simulink model "simThreeLinkFTC"  (R2014b)
settings: Solver=ode45  StartTime=0.0  StopTime=tof  FixedStep=dt  MaxStep=dtmax  RelTol=1e-3
values from neighbouring files (symbols this model uses):
  alpha = 1    [robotArmWith2Links.m]    (also in threeLinkFTC.m; twoLinkFTC.m; twoLinkFTCwAdaptive.m)
  Ar = [0 5; -30 -30]    [robotArmWith2Links.m]    (also in threeLinkFTC.m = [0 1; -5 -5]; twoLinkFTC.m = [0 10; -40 -40]; twoLinkFTCwAdaptive.m = [0 5; -250 -250])
  Arm1 = [0 1; -wn^2 -2*ksi*wn]    [robotArmWith2Links.m]    (also in threeLinkFTC.m; twoLinkFTC.m; twoLinkFTCwAdaptive.m)
  As = zeros(nofstates,nofstates)    [threeLinkFTC.m]    (also in twoLinkFDIbasisComparison.m; twoLinkFTC.m; twoLinkFTCwAdaptive.m)
  Brm1 = [0 wn^2]'    [robotArmWith2Links.m]    (also in threeLinkFTC.m; twoLinkFTC.m; twoLinkFTCwAdaptive.m)
  Dhat0 = zeros(6,1)    [threeLinkFTC.m]    (also in twoLinkFDIbasisComparison.m = zeros(4,1); twoLinkFTC.m = zeros(4,1); twoLinkFTCwAdaptive.m = zeros(4,1))
  Dlimit = 10    [threeLinkFTC.m]    (also in twoLinkFTC.m; twoLinkFTCwAdaptive.m)
  dtFc = 1*dtmax    (= 0.001)    [threeLinkFTC.m]    (also in twoLinkFDIbasisComparison.m; twoLinkFTC.m; twoLinkFTCwAdaptive.m)
  epsilon = 0.5    [robotArmWith2Links.m]    (also in threeLinkFTC.m; twoLinkFTC.m; twoLinkFTCwAdaptive.m)
  epsilontheta = 0.01    [threeLinkFTC.m]    (also in twoLinkFDIbasisComparison.m; twoLinkFTC.m; twoLinkFTCwAdaptive.m)
  faultyArm = 3    [threeLinkFTC.m]    (also in twoLinkFDIbasisComparison.m = 2; twoLinkFTC.m = 2; twoLinkFTCwAdaptive.m = 1)
  FDstart = 0.5    [threeLinkFTC.m]    (also in twoLinkFTC.m; twoLinkFTCwAdaptive.m)
  fmPosition = [0 90 -45]'*pi/180    [threeLinkFTC.m]    (also in twoLinkFTC.m = [90 0]'*pi/180; twoLinkFTCwAdaptive.m = [90 0]'*pi/180)
  g = 9.81    [robotArmWith2Links.m]    (also in threeLinkFTC.m; twoLinkFDIbasisComparison.m; twoLinkFTC.m; twoLinkFTCwAdaptive.m)
  GammaW = 1000    [threeLinkFTC.m]    (also in twoLinkFDIbasisComparison.m; twoLinkFTC.m; twoLinkFTCwAdaptive.m)
  I1 = 8.33e-2    (= 0.0833)    [robotArmWith2Links.m]    (also in threeLinkFTC.m = 0.0833333333333; twoLinkFDIbasisComparison.m = 0.0833333333333; twoLinkFTC.m = 0.0833333333333; twoLinkFTCwAdaptive.m = 0.0833333333333)
  I2 = 8.33e-2    (= 0.0833)    [robotArmWith2Links.m]    (also in threeLinkFTC.m = 0.0833333333333; twoLinkFDIbasisComparison.m = 0.0833333333333; twoLinkFTC.m = 0.0833333333333; twoLinkFTCwAdaptive.m = 0.0833333333333)
  I3 = m3*l3^2*1/12    (= 0.0833333333333)    [threeLinkFTC.m]
  ifault = 2    [threeLinkFTC.m]    (also in twoLinkFDIbasisComparison.m; twoLinkFTC.m; twoLinkFTCwAdaptive.m)
  K1 = 2*wn*ksi    (= 87.9645943005)    [robotArmWith2Links.m]    (also in threeLinkFTC.m = 8.79645943005; twoLinkFTC.m; twoLinkFTCwAdaptive.m = 43.9822971503)
  K2 = wn^2    (= 986.960440109)    [robotArmWith2Links.m]    (also in threeLinkFTC.m = 39.4784176044; twoLinkFTC.m; twoLinkFTCwAdaptive.m)
  Kp = wn^2    (= 157.913670417)    [threeLinkFTC.m]    (also in twoLinkFDIbasisComparison.m = 3947.84176044; twoLinkFTC.m = 3947.84176044; twoLinkFTCwAdaptive.m = 3947.84176044)
  Kv = 2*ksi*wn    (= 17.5929188601)    [threeLinkFTC.m]    (also in twoLinkFDIbasisComparison.m = 125.663706144; twoLinkFTC.m = 125.663706144; twoLinkFTCwAdaptive.m = 125.663706144)
  l1 = 1    [robotArmWith2Links.m]    (also in threeLinkFTC.m; twoLinkFDIbasisComparison.m; twoLinkFTC.m; twoLinkFTCwAdaptive.m)
  l2 = 1    [robotArmWith2Links.m]    (also in threeLinkFTC.m; twoLinkFDIbasisComparison.m; twoLinkFTC.m; twoLinkFTCwAdaptive.m)
  lc1 = l1/2    (= 0.5)    [robotArmWith2Links.m]    (also in threeLinkFTC.m; twoLinkFDIbasisComparison.m; twoLinkFTC.m; twoLinkFTCwAdaptive.m)
  lc2 = l2/2    (= 0.5)    [robotArmWith2Links.m]    (also in threeLinkFTC.m; twoLinkFDIbasisComparison.m; twoLinkFTC.m; twoLinkFTCwAdaptive.m)
  m1 = 1    [robotArmWith2Links.m]    (also in threeLinkFTC.m; twoLinkFDIbasisComparison.m; twoLinkFTC.m; twoLinkFTCwAdaptive.m)
  m2 = 1    [robotArmWith2Links.m]    (also in threeLinkFTC.m; twoLinkFDIbasisComparison.m; twoLinkFTC.m; twoLinkFTCwAdaptive.m)
  m3 = 1    [threeLinkFTC.m]
  nCheby = 4    [threeLinkFTC.m]    (also in twoLinkFDIbasisComparison.m; twoLinkFTC.m; twoLinkFTCwAdaptive.m)
  Ps = lyap(As(4:6,4:6)',Q)    [threeLinkFTC.m]    (also in twoLinkFDIbasisComparison.m = lyap(As(3:4,3:4)',Q); twoLinkFTC.m = lyap(As(3:4,3:4)',Q); twoLinkFTCwAdaptive.m = lyap(As(3:4,3:4)',Q))
  q0 = [80 20]'*pi/180    [robotArmWith2Links.m]    (also in threeLinkFTC.m = [90 0 0]'*pi/180; twoLinkFDIbasisComparison.m = [90 0]'*pi/180; twoLinkFTC.m = [90 0]'*pi/180; twoLinkFTCwAdaptive.m = [90 0]'*pi/180)
  qdot0 = [0 0]'    [robotArmWith2Links.m]    (also in threeLinkFTC.m = [0 0 0]'*pi/180; twoLinkFDIbasisComparison.m = [0 0]'*pi/180; twoLinkFTC.m = [0 0]'*pi/180; twoLinkFTCwAdaptive.m = [0 0]'*pi/180)
  r0 = [0 0]'    [robotArmWith2Links.m]    (also in threeLinkFTC.m; twoLinkFTC.m; twoLinkFTCwAdaptive.m)
  rmax = inf*[50*pi/180 inf]'    [robotArmWith2Links.m]    (also in threeLinkFTC.m; twoLinkFTC.m; twoLinkFTCwAdaptive.m)
  rmin = -rmax    [robotArmWith2Links.m]    (also in threeLinkFTC.m; twoLinkFTC.m; twoLinkFTCwAdaptive.m)
  tfault = 5    [threeLinkFTC.m]    (also in twoLinkFDIbasisComparison.m; twoLinkFTC.m; twoLinkFTCwAdaptive.m = 1)
  W0 = 0    [threeLinkFTC.m]    (also in twoLinkFDIbasisComparison.m; twoLinkFTC.m; twoLinkFTCwAdaptive.m)
  Wbnd = 1000    [threeLinkFTC.m]    (also in twoLinkFDIbasisComparison.m; twoLinkFTC.m; twoLinkFTCwAdaptive.m)
  xhat0 = [q0 ; qdot0]    [threeLinkFTC.m]    (also in twoLinkFDIbasisComparison.m; twoLinkFTC.m; twoLinkFTCwAdaptive.m)
undefined symbols (not defined in the file or in its folder): Intmax, Intmin
libraries: simulink x9, vrlib x3, dspbuff3 x1
(part 1 of 3)
settings Model: Creator=alp.marangoz  LastModifiedBy=alpmarangoz
settings SolverCC: AutoInsertRateTranBlk=on
settings DataIOCC: SignalLoggingSaveFormat=ModelDataLogs
settings OptimizationCC: ExpressionDepthLimit=2147483647
settings DebuggingCC: UnderspecifiedInitializationDetection=Classic  MergeDetectMultiDrivingBlocksExec=none  InheritedTsInSrcMsg=none  CheckMatrixSingularityMsg=error  FcnCallInpInsideContextMsg=UseLocalSettings  StateNameClashWarn=warning
settings GRTTargetCC: CombineOutputUpdateFcns=off  GRTInterface=on

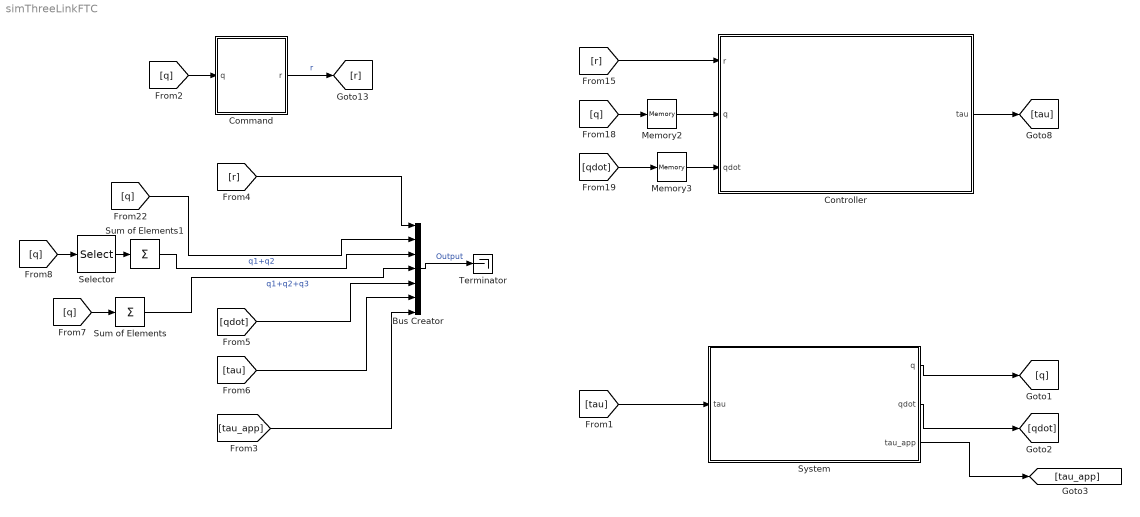
== system simThreeLinkFTC ==
  Bus Creator : BusCreator  Inputs=7
  Command : Subsystem  TreatAsAtomicUnit=on  SystemSampleTime=dtFc
  Controller : Subsystem  TreatAsAtomicUnit=on  SystemSampleTime=dtFc
  Memory2 : Memory  X0=q0  InheritSampleTime=on  LinearizeMemory=on  LinearizeAsDelay=on
  Memory3 : Memory  X0=qdot0  InheritSampleTime=on  LinearizeMemory=on  LinearizeAsDelay=on
  Selector : Selector  InputPortWidth=3  Indices=[1 2]
  Sum of Elements : Sum  Inputs=+
  Sum of Elements1 : Sum  Inputs=+
  System : Subsystem  TreatAsAtomicUnit=on
  Terminator : Terminator
  wires:
  Command/1(r) -> [r]  "r"
  [r] -> Controller/1(r)
  Controller/1(tau) -> [tau]
  [tau] -> System/1(tau)
  [q] -> Memory2/1
  [qdot] -> Memory3/1
  System/1(q) -> [q]
  System/2(qdot) -> [qdot]
  [q] -> Command/1(q)
  Memory2/1 -> Controller/2(q)
  Memory3/1 -> Controller/3(qdot)
  Bus Creator/1 -> Terminator/1  "Output"
  [r] -> Bus Creator/1
  [q] -> Bus Creator/2
  [qdot] -> Bus Creator/5
  [tau] -> Bus Creator/6
  System/3(tau_app) -> [tau_app]
  [tau_app] -> Bus Creator/7
  [q] -> Selector/1
  Selector/1 -> Sum of Elements1/1
  Sum of Elements1/1 -> Bus Creator/3  "q1+q2"
  [q] -> Sum of Elements/1
  Sum of Elements/1 -> Bus Creator/4  "q1+q2+q3"

== system simThreeLinkFTC/Command ==
  q : Inport
  Add1 : Sum  Inputs=-+
  From Workspace : FromWorkspace  VariableName=r  Interpolate=off  OutputAfterFinalValue=Setting to zero
  Memory2 : Memory  X0=q0  InheritSampleTime=on  LinearizeMemory=on  LinearizeAsDelay=on
  Reshape1 : Reshape  OutputDimensionality=Column vector (2-D)
  Terminator1 : Terminator
  r : Outport  InitialOutput=0
  wires:
  From Workspace/1 -> Reshape1/1
  Reshape1/1 -> r/1, [r]  "r"
  [r] -> Add1/2
  Add1/1 -> Terminator1/1  "e"
  [q] -> Add1/1  "q"
  q/1 -> Memory2/1  "q"
  Memory2/1 -> [q]

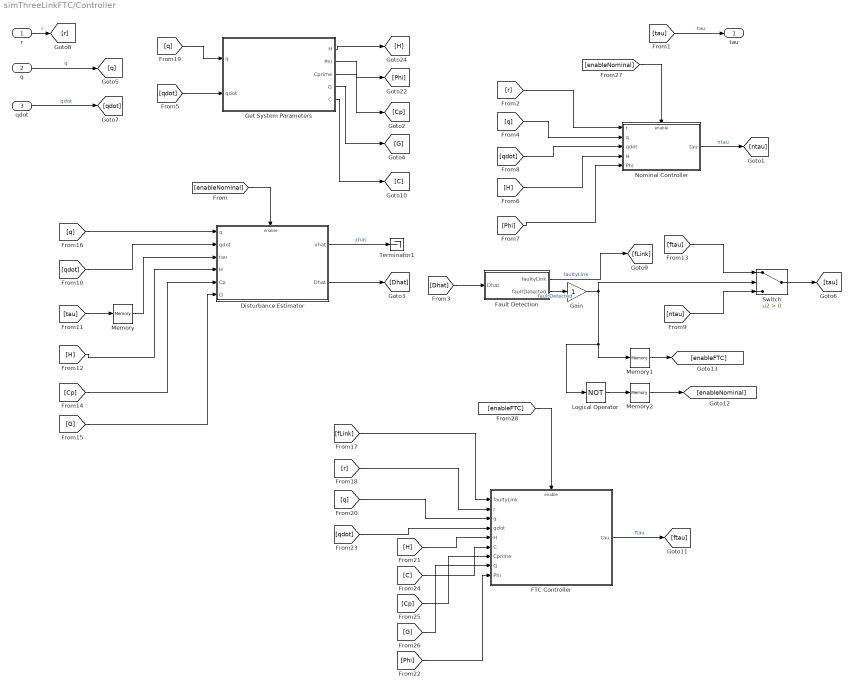
== system simThreeLinkFTC/Controller ==
  r : Inport
  q : Inport  Port=2
  qdot : Inport  Port=3
  Disturbance Estimator : Subsystem
  FTC Controller : Subsystem
  Fault Detection : Subsystem  TreatAsAtomicUnit=on
  Gain : Gain
  Get System Parameters : Subsystem
  Logical Operator : Logic  Operator=NOT  AllPortsSameDT=off  OutDataTypeStr=boolean
  Memory : Memory  InheritSampleTime=on  LinearizeMemory=on  LinearizeAsDelay=on
  Memory1 : Memory  InheritSampleTime=on  LinearizeMemory=on  LinearizeAsDelay=on
  Memory2 : Memory  InheritSampleTime=on  LinearizeMemory=on  LinearizeAsDelay=on
  Nominal Controller : Subsystem
  Switch : Switch  Criteria=u2 > Threshold
  Terminator1 : Terminator
  tau : Outport
  wires:
  r/1 -> [r]  "r"
  qdot/1 -> [qdot]  "qdot"
  q/1 -> [q]  "q"
  [tau] -> tau/1  "tau"
  [q] -> Get System Parameters/1(q)
  Nominal Controller/1(tau) -> [ntau]  "ntau"
  [r] -> Nominal Controller/1(r)
  [H] -> Nominal Controller/4(H)
  [Phi] -> Nominal Controller/5(Phi)
  [qdot] -> Get System Parameters/2(qdot)
  Get System Parameters/1(H) -> [H]
  Get System Parameters/2(Phi) -> [Phi]
  Get System Parameters/3(Cprime) -> [Cp]
  [q] -> Disturbance Estimator/1(q)
  [qdot] -> Disturbance Estimator/2(qdot)
  [H] -> Disturbance Estimator/4(H)
  [Cp] -> Disturbance Estimator/5(Cp)
  [G] -> Disturbance Estimator/6(G)
  Disturbance Estimator/1(xhat) -> Terminator1/1  "xhat"
  Disturbance Estimator/2(Dhat) -> [Dhat]
  [qdot] -> Nominal Controller/3(qdot)
  [q] -> Nominal Controller/2(q)
  [tau] -> Memory/1
  Get System Parameters/4(G) -> [G]
  [Dhat] -> Fault Detection/1(Dhat)
  Switch/1 -> [tau]
  Fault Detection/2(faultDetected) -> Gain/1  "faultDetected"
  [ntau] -> Switch/3
  [ftau] -> Switch/1
  Fault Detection/1(faultyLink) -> [fLink]  "faultyLink"
  Get System Parameters/5(C) -> [C]
  FTC Controller/1(tau) -> [ftau]  "ftau"
  [H] -> FTC Controller/5(H)
  [C] -> FTC Controller/6(C)
  [Cp] -> FTC Controller/7(Cprime)
  [G] -> FTC Controller/8(G)
  [qdot] -> FTC Controller/4(qdot)
  [q] -> FTC Controller/3(q)
  [Phi] -> FTC Controller/9(Phi)
  [r] -> FTC Controller/2(r)
  [fLink] -> FTC Controller/1(faultyLink)
  Memory/1 -> Disturbance Estimator/3(tau)
  [enableNominal] -> Disturbance Estimator/Enable
  [enableNominal] -> Nominal Controller/Enable
  Logical Operator/1 -> Memory2/1
  [enableFTC] -> FTC Controller/Enable
  Memory1/1 -> [enableFTC]
  Memory2/1 -> [enableNominal]
  Gain/1 -> Switch/2, Logical Operator/1, Memory1/1

== system simThreeLinkFTC/System ==
  tau : Inport
  Fault Insertion : Subsystem
  Integration : Subsystem  TreatAsAtomicUnit=on
  Memory2 : Memory  X0=q0  InheritSampleTime=on  LinearizeMemory=on  LinearizeAsDelay=on
  Memory4 : Memory  X0=qdot0  InheritSampleTime=on  LinearizeMemory=on  LinearizeAsDelay=on
  Reshape5 : Reshape  OutputDimensionality=Column vector (2-D)
  System Parameters : Subsystem
  q : Outport
  qdot : Outport  Port=2
  tau_app : Outport  Port=3
  wires:
  [q] -> Memory2/1
  [qdot] -> Memory4/1
  tau/1 -> Reshape5/1  "tau"
  Reshape5/1 -> [tau]  "tau"
  [q] -> q/1  "q"
  [qdot] -> qdot/1  "qdot"
  Memory4/1 -> System Parameters/2(qdot)
  [H] -> Integration/1(H)
  [C] -> Integration/2(C)
  [tau_app] -> Integration/4(tau)
  [lockJoint] -> Integration/5(lockJoint)
  [G] -> Integration/3(G)
  Integration/1(q) -> [q]
  Integration/2(qdot) -> [qdot]
  Memory2/1 -> System Parameters/1(q)
  Fault Insertion/2(lockJoint) -> [lockJoint]
  Fault Insertion/1(tau_app) -> [tau_app]
  [tau] -> Fault Insertion/1(tau)
  [tau_app] -> tau_app/1  "tau_app"
  System Parameters/1(H) -> [H]
  System Parameters/2(C) -> [C]
  System Parameters/3(G) -> [G]

== system simThreeLinkFTC/Controller/Disturbance Estimator ==
  q : Inport
  qdot : Inport  Port=2
  tau : Inport  Port=3
  H : Inport  Port=4
  Cp : Inport  Port=5
  G : Inport  Port=6
  Enable : EnablePort
  Memory1 : Memory  X0=Dhat0  InheritSampleTime=on  LinearizeMemory=on
  Product3 : Product  Inputs=/  Multiplication=Matrix(*)  RndMeth=Zero
  State Error Calculation : Subsystem
  getDisturbance : Subsystem
  getx : Subsystem
  getxhat : Subsystem
  xhat : Outport  InitialOutput=xhat0
  Dhat : Outport  Port=2
  wires:
  getx/2(xdot) -> [xdot]
  [qdot] -> getx/2(qdot)
  [q] -> getx/1(q)
  Cp/1 -> [Cp]
  Product3/1 -> [Hinv]
  H/1 -> [H], Product3/1
  tau/1 -> [tau]
  [xhat] -> xhat/1
  q/1 -> [q]
  qdot/1 -> [qdot]
  getx/1(x) -> [x]  "x"
  [H] -> getx/3(H)
  [Hinv] -> getxhat/1(Hinv)
  [tau] -> getxhat/2(tau)
  [Cp] -> getxhat/3(Cp)
  [es] -> getxhat/5(es)
  [Dhat] -> Memory1/1
  G/1 -> [G]
  getxhat/1(xhat) -> [xhat]  "xhat"
  getxhat/2(xhatdot) -> [xhatdot]
  [x] -> State Error Calculation/1(x)
  [xdot] -> State Error Calculation/2(xdot)
  [xhat] -> State Error Calculation/3(xhat)
  [xhatdot] -> State Error Calculation/4(xhatdot)
  [Hinv] -> State Error Calculation/5(Hinv)
  State Error Calculation/1(es) -> [es]
  [xhat] -> getDisturbance/1(x)
  [tau] -> getDisturbance/2(tau)
  [es] -> getDisturbance/3(es)
  getDisturbance/1(Dhat) -> [Dhat]
  [Dhat] -> Dhat/1
  Memory1/1 -> getxhat/6(Dhat)
  [G] -> getxhat/4(G)

== system simThreeLinkFTC/Controller/FTC Controller ==
  faultyLink : Inport
  r : Inport  Port=2
  q : Inport  Port=3
  qdot : Inport  Port=4
  H : Inport  Port=5
  C : Inport  Port=6
  Cprime : Inport  Port=7
  G : Inport  Port=8
  Phi : Inport  Port=9
  Enable : EnablePort
  1st Link Compensator : Subsystem  TreatAsAtomicUnit=on  SystemSampleTime=dtFc
  3rd Link Compensator : Subsystem  TreatAsAtomicUnit=on  SystemSampleTime=dtFc
  Compare To Constant : simulink/Logic and Bit Operations/Compare To Constant  relop===  const=3.0  OutDataTypeStr=boolean
  Compare To Constant1 : simulink/Logic and Bit Operations/Compare To Constant  relop===  const=1  OutDataTypeStr=boolean
  Constant : Constant  Value=fmPosition  VectorParams1D=off
  Gain1 : Gain  Gain=[1 2 3]  Multiplication=Matrix(K*u)
  Ground : Ground
  Multiport Switch : MultiPortSwitch
  Terminator1 : Terminator
  Terminator6 : Terminator
  Terminator8 : Terminator
  tau : Outport
  wires:
  [tau] -> tau/1  "tau"
  faultyLink/1 -> Gain1/1
  Cprime/1 -> Terminator6/1
  G/1 -> [G]
  Phi/1 -> Terminator8/1
  q/1 -> [q]
  qdot/1 -> [qdot]
  H/1 -> [H]
  C/1 -> [C]
  r/1 -> Terminator1/1  "r"
  Constant/1 -> [qc]
  [H] -> 3rd Link Compensator/4(H)
  [G] -> 3rd Link Compensator/6(G)
  [qdot] -> 3rd Link Compensator/3(qdot)
  [C] -> 3rd Link Compensator/5(C)
  [q] -> 3rd Link Compensator/2(q)
  [qc] -> 3rd Link Compensator/1(qc)
  [H] -> 1st Link Compensator/4(H)
  [G] -> 1st Link Compensator/6(G)
  [qdot] -> 1st Link Compensator/3(qdot)
  [C] -> 1st Link Compensator/5(C)
  [q] -> 1st Link Compensator/2(q)
  [qc] -> 1st Link Compensator/1(qc)
  3rd Link Compensator/1(tau) -> [tau_3comp]  "tau3_comp"
  1st Link Compensator/1(tau) -> [tau_1comp]  "tau1_comp"
  Multiport Switch/1 -> [tau]  "tau"
  [tau_3comp] -> Multiport Switch/4
  Ground/1 -> Multiport Switch/3
  [tau_1comp] -> Multiport Switch/2
  Gain1/1 -> [faultyArm]  "faultyArm"
  [faultyArm] -> Multiport Switch/1
  [faultyArm] -> Compare To Constant/1
  Compare To Constant/1 -> 3rd Link Compensator/Enable
  [faultyArm] -> Compare To Constant1/1
  Compare To Constant1/1 -> 1st Link Compensator/Enable

== system simThreeLinkFTC/Controller/Fault Detection ==
  Dhat : Inport
  Abs : Abs
  Compare To Constant : simulink/Logic and Bit Operations/Compare To Constant  relop=>=  const=Dlimit  OutDataTypeStr=boolean
  Compare To Constant1 : simulink/Logic and Bit Operations/Compare To Constant  relop=>=  const=FDstart  OutDataTypeStr=boolean
  Digital Clock : DigitalClock  SampleTime=-1
  Logical Operator : Logic  AllPortsSameDT=off  OutDataTypeStr=boolean
  Select 3 : Selector  NumberOfDimensions=2  InputPortWidth=3  IndexOptions=Index vector (dialog),Index vector (dialog)  Indices=[4 5 6],1  OutputSizes=1,1
  Sum of Elements : Sum  Inputs=+
  Triggered step : Subsystem
  faultyLink : Outport
  faultDetected : Outport  Port=2
  wires:
  Dhat/1 -> Select 3/1
  Abs/1 -> Compare To Constant/1
  Select 3/1 -> Abs/1
  Compare To Constant/1 -> Sum of Elements/1, faultyLink/1
  Triggered step/1(Out1) -> faultDetected/1
  Sum of Elements/1 -> Logical Operator/1
  Logical Operator/1 -> Triggered step/Trigger
  Digital Clock/1 -> Compare To Constant1/1
  Compare To Constant1/1 -> Logical Operator/2

== system simThreeLinkFTC/Controller/Get System Parameters ==
  q : Inport
  qdot : Inport  Port=2
  Constant : Constant  Value=I1+m1*lc1^2+m2*l1^2+m3*l1^2  VectorParams1D=off
  Constant2 : Constant  Value=[0 0 0]'  VectorParams1D=off
  Constant3 : Constant  Value=I2+I3+m2*lc2^2+m3*l2^2  VectorParams1D=off
  Constant4 : Constant  Value=m2*l1*lc2+m3*l1*l2  VectorParams1D=off
  Constant5 : Constant  Value=I3  VectorParams1D=off
  Product5 : Product  Multiplication=Matrix(*)  RndMeth=Zero
  Sum of Elements1 : Sum
  Terminator18 : Terminator
  get Plant Parameters : Subsystem
  getC : Subsystem
  getCprime : Subsystem
  getH : Subsystem
  H : Outport
  Phi : Outport  Port=2
  Cprime : Outport  Port=3
  G : Outport  Port=4
  C : Outport  Port=5
  wires:
  q/1 -> [q]
  qdot/1 -> [qdot]
  getH/1(H) -> [H]
  Constant2/1 -> [G]
  [C] -> Product5/1
  [qdot] -> Product5/2
  Product5/1 -> Sum of Elements1/1
  [G] -> Sum of Elements1/2
  Sum of Elements1/1 -> [Phi]  "Phi"
  [H] -> H/1
  [Phi] -> Phi/1
  [Cprime] -> Cprime/1
  Constant/1 -> [alpha]
  [G] -> G/1
  get Plant Parameters/1(busData) -> Terminator18/1  "system"
  [C] -> get Plant Parameters/2(C)
  [H] -> get Plant Parameters/1(H)
  [G] -> get Plant Parameters/3(G)
  [qdot] -> get Plant Parameters/4(qdot)
  [Cprime] -> get Plant Parameters/5(Cprime)
  [C] -> C/1
  Constant3/1 -> [beta]
  Constant4/1 -> [gamma]
  Constant5/1 -> [delta]
  [alpha] -> getH/2(alpha)
  [beta] -> getH/3(beta)
  [gamma] -> getH/4(gamma)
  [delta] -> getH/5(delta)
  [q] -> getH/1(q)
  getC/1(C) -> [C]
  [alpha] -> getC/3(alpha)
  [beta] -> getC/4(beta)
  [gamma] -> getC/5(gamma)
  [delta] -> getC/6(delta)
  [q] -> getC/1(q)
  [qdot] -> getC/2(qdot)
  getCprime/1(Cprime) -> [Cprime]
  [alpha] -> getCprime/3(alpha)
  [beta] -> getCprime/4(beta)
  [gamma] -> getCprime/5(gamma)
  [delta] -> getCprime/6(delta)
  [q] -> getCprime/1(q)
  [qdot] -> getCprime/2(qdot)

== system simThreeLinkFTC/Controller/Nominal Controller ==
  r : Inport
  q : Inport  Port=2
  qdot : Inport  Port=3
  H : Inport  Port=4
  Phi : Inport  Port=5
  Enable : EnablePort
  FBL Controller : Subsystem
  Saturation : Saturate  UpperLimit=2000  LowerLimit=-2000
  tau : Outport
  wires:
  r/1 -> [r]  "r"
  Phi/1 -> [Phi]
  H/1 -> [H]
  [tau] -> Saturation/1  "tau"
  [r] -> FBL Controller/1(r)
  [H] -> FBL Controller/4(H)
  [Phi] -> FBL Controller/5(Phi)
  Saturation/1 -> tau/1
  FBL Controller/1(tau) -> [tau]
  q/1 -> [q]
  qdot/1 -> [qdot]
  [qdot] -> FBL Controller/3(qdot)
  [q] -> FBL Controller/2(q)

== system simThreeLinkFTC/System/Fault Insertion ==
  tau : Inport
  Clock : Clock
  Compare To Constant : simulink/Logic and Bit Operations/Compare To Constant  relop===  const=faultyArm  OutDataTypeStr=boolean
  Compare To Constant1 : simulink/Logic and Bit Operations/Compare To Constant  relop===  const=3  OutDataTypeStr=uint8  ZeroCross=off
  Constant1 : Constant  Value=ifault  VectorParams1D=off
  Constant2 : Constant  Value=[ 1 1 1]'
  Constant4 : Constant  Value=tfault
  Constant5 : Constant  Value=[1 2 3]'  VectorParams1D=off
  Data Type Conversion : DataTypeConversion
  Data Type Conversion1 : DataTypeConversion
  Ground2 : Ground
  Logical Operator1 : Logic  Operator=NOT  AllPortsSameDT=off  OutDataTypeStr=boolean
  Logical Operator2 : Logic  AllPortsSameDT=off  OutDataTypeStr=boolean
  MinMax1 : MinMax  Function=max  Inputs=2
  Product : Product
  Sign : Signum
  Subtract1 : Sum  Inputs=+-
  Switch2 : Switch  Criteria=u2 > Threshold
  Switch3 : Switch  Criteria=u2 > Threshold
  tau_app : Outport
  lockJoint : Outport  Port=2
  wires:
  Clock/1 -> [time]
  MinMax1/1 -> [faultInsertion]  "faultInsertion"
  Sign/1 -> MinMax1/1
  Ground2/1 -> MinMax1/2
  Subtract1/1 -> Sign/1
  Constant4/1 -> Subtract1/2
  [time] -> Subtract1/1
  tau/1 -> [tau]  "tau"
  Constant1/1 -> Compare To Constant1/1
  Data Type Conversion1/1 -> [lockJoint]
  [faultInsertion] -> Switch2/2
  [faultytau] -> Switch2/1
  [tau] -> Switch2/3
  Switch2/1 -> tau_app/1  "tau_app"
  [faultyJoint] -> Switch3/1
  Constant2/1 -> Switch3/3
  Switch3/1 -> lockJoint/1  "lockJoint"
  Compare To Constant1/1 -> Data Type Conversion1/1
  Compare To Constant/1 -> Logical Operator1/1
  Constant5/1 -> Compare To Constant/1
  Logical Operator1/1 -> Data Type Conversion/1
  Data Type Conversion/1 -> [faultyJoint]
  Product/1 -> [faultytau]
  [faultyJoint] -> Product/1
  [tau] -> Product/2
  [faultInsertion] -> Logical Operator2/1
  [lockJoint] -> Logical Operator2/2
  Logical Operator2/1 -> Switch3/2

== system simThreeLinkFTC/System/Integration ==
  H : Inport
  C : Inport  Port=2
  G : Inport  Port=3
  tau : Inport  Port=4
  lockJoint : Inport  Port=5
  Add : Sum  Inputs=+-
  Constant1 : Constant  Value=2*pi
  Integrator2 : Integrator  InitialCondition=qdot0
  Integrator3 : Integrator  InitialCondition=q0
  Math Function1 : Math  Operator=rem  SaturateOnIntegerOverflow=on
  Product1 : Product  RndMeth=Zero
  Product3 : Product  RndMeth=Zero
  Product4 : Product  Multiplication=Matrix(*)  RndMeth=Zero
  Product5 : Product  Multiplication=Matrix(*)  RndMeth=Zero
  Product6 : Product  Multiplication=Matrix(*)  RndMeth=Zero
  Product7 : Product  Inputs=/  Multiplication=Matrix(*)  RndMeth=Zero
  Reshape : Reshape  OutputDimensionality=Column vector (2-D)
  Reshape3 : Reshape  OutputDimensionality=Column vector (2-D)
  Sum : Sum  Inputs=|+-
  q : Outport
  qdot : Outport  Port=2
  wires:
  lockJoint/1 -> [lockJoint]
  tau/1 -> [tau]
  C/1 -> [C]
  H/1 -> Product7/1
  [qdot] -> qdot/1  "qdot"
  [q] -> q/1  "q"
  G/1 -> [G]
  [G] -> Add/2
  [Hinv] -> Product4/1
  Add/1 -> Product4/2
  Product4/1 -> Sum/1
  [Hinv] -> Product5/1
  [C] -> Product5/2
  Product5/1 -> Product6/1
  Product6/1 -> Sum/2
  Integrator3/1 -> Reshape3/1
  Reshape/1 -> Product6/2, Integrator3/1, [qdot]
  Reshape3/1 -> Math Function1/1
  Product7/1 -> [Hinv]
  [tau] -> Add/1  "tau_app"
  Constant1/1 -> Math Function1/2
  Math Function1/1 -> [q]  "qr"
  Sum/1 -> Product3/2
  Product3/1 -> Integrator2/1  "qddot"
  [lockJoint] -> Product3/1, Product1/1
  Integrator2/1 -> Product1/2
  Product1/1 -> Reshape/1  "qdot"

== system simThreeLinkFTC/System/System Parameters ==
  q : Inport
  qdot : Inport  Port=2
  Constant : Constant  Value=I1+m1*lc1^2+m2*l1^2+m3*l1^2  VectorParams1D=off
  Constant2 : Constant  Value=[0 0 0]'  VectorParams1D=off
  Constant3 : Constant  Value=I2+I3+m2*lc2^2+m3*l2^2  VectorParams1D=off
  Constant4 : Constant  Value=m2*l1*lc2+m3*l1*l2  VectorParams1D=off
  Constant5 : Constant  Value=I3  VectorParams1D=off
  Terminator18 : Terminator
  get Plant Parameters : Subsystem
  getC : Subsystem
  getH : Subsystem
  H : Outport
  C : Outport  Port=2
  G : Outport  Port=3
  wires:
  q/1 -> [q]
  qdot/1 -> [qdot]
  getH/1(H) -> [H]
  Constant2/1 -> [G]
  [H] -> H/1
  Constant/1 -> [alpha]
  [G] -> G/1
  get Plant Parameters/1(busData) -> Terminator18/1  "system"
  [C] -> get Plant Parameters/2(C)
  [H] -> get Plant Parameters/1(H)
  [G] -> get Plant Parameters/3(G)
  [qdot] -> get Plant Parameters/4(qdot)
  [C] -> C/1
  Constant3/1 -> [beta]
  Constant4/1 -> [gamma]
  Constant5/1 -> [delta]
  [alpha] -> getH/2(alpha)
  [beta] -> getH/3(beta)
  [gamma] -> getH/4(gamma)
  [delta] -> getH/5(delta)
  [q] -> getH/1(q)
  getC/1(C) -> [C]
  [alpha] -> getC/3(alpha)
  [beta] -> getC/4(beta)
  [gamma] -> getC/5(gamma)
  [delta] -> getC/6(delta)
  [q] -> getC/1(q)
  [qdot] -> getC/2(qdot)
  [alpha] -> get Plant Parameters/5(alpha)
  [beta] -> get Plant Parameters/6(beta)
  [gamma] -> get Plant Parameters/7(gamma)
  [delta] -> get Plant Parameters/8(delta)

== system simThreeLinkFTC/Controller/Disturbance Estimator/State Error Calculation ==
  x : Inport
  xdot : Inport  Port=2
  xhat : Inport  Port=3
  xhatdot : Inport  Port=4
  Hinv : Inport  Port=5
  Add : Sum  Inputs=+-
  Add1 : Sum  Inputs=+-
  Discrete Derivative1 : simulink/Discrete/Discrete Derivative  gainval=1.0  ICPrevScaledInput=0.0  InputProcessing=Inherited  OutMin=[]  OutMax=[]  OutDataType=fixdt(1, 16)  OutScaling=2^-10  RndMeth=Round  DoSatur=off
  Memory1 : Memory  X0=xhat0  InheritSampleTime=on  LinearizeMemory=on  LinearizeAsDelay=on
  Memory4 : Memory  X0=xhat0  InheritSampleTime=on  LinearizeMemory=on  LinearizeAsDelay=on
  Product6 : Product  Multiplication=Matrix(*)  RndMeth=Zero
  Reshape1 : Reshape  OutputDimensionality=Column vector (2-D)
  Reshape2 : Reshape  OutputDimensionality=Column vector (2-D)
  Reshape3 : Reshape  OutputDimensionality=Column vector (2-D)
  Saturation : Saturate  UpperLimit=10  LowerLimit=-10  ZeroCross=off
  Terminator{1..4} (4 alike) : Terminator
  "[1 2 3]" : Selector  NumberOfDimensions=2  InputPortWidth=3  IndexOptions=Index vector (dialog),Index vector (dialog)  Indices=[1 2 3],1  OutputSizes=1,1
  "[4 5 6]" : Selector  NumberOfDimensions=2  InputPortWidth=3  IndexOptions=Index vector (dialog),Index vector (dialog)  Indices=[4 5 6],1  OutputSizes=1,1
  es : Outport
  wires:
  [Hinv] -> Product6/1
  xdot/1 -> [xdot]
  x/1 -> [x]
  Saturation/1 -> [esdot]  "esdotflt"
  Discrete Derivative1/1 -> Saturation/1  "esdot"
  Reshape2/1 -> [es], Discrete Derivative1/1
  [xhat] -> Memory4/1
  [x] -> Add/2
  Add/1 -> Reshape2/1  "es"
  Memory4/1 -> Add/1
  xhat/1 -> [xhat]
  xhatdot/1 -> [xhatdot]
  Hinv/1 -> [Hinv]
  [xhatdot] -> Memory1/1
  [xdot] -> Add1/2
  Add1/1 -> Reshape1/1  "esdot2"
  Memory1/1 -> Add1/1
  [esdot] -> Terminator3/1
  [es] -> es/1
  [xhat] -> Reshape3/1
  Reshape3/1 -> "[1 2 3]"/1, "[4 5 6]"/1
  "[4 5 6]"/1 -> Product6/2
  "[1 2 3]"/1 -> Terminator2/1  "qhat"
  Product6/1 -> Terminator1/1  "qhatdot"
  Reshape1/1 -> Terminator4/1

== system simThreeLinkFTC/Controller/Disturbance Estimator/getDisturbance ==
  x : Inport
  tau : Inport  Port=2
  es : Inport  Port=3
  Chebyshev Basis Functions : Subsystem
  Constant : Constant  Value=[0 0 0]'  VectorParams1D=off
  Gain : Gain
  Gain1 : Gain
  Mux1 : Mux  Inputs=2
  Reshape1 : Reshape  OutputDimensionality=Column vector (2-D)
  "[4 5 6]" : Selector  NumberOfDimensions=2  InputPortWidth=3  IndexOptions=Index vector (dialog),Index vector (dialog)  Indices=[4 5 6],1  OutputSizes=1,1
  getDhat : Subsystem  TreatAsAtomicUnit=on
  Dhat : Outport
  wires:
  [Dhat] -> Dhat/1  "Dhat"
  x/1 -> [x]
  tau/1 -> [tau]
  es/1 -> [es]
  [es] -> "[4 5 6]"/1
  "[4 5 6]"/1 -> [es34]
  [Dhat12] -> Gain/1
  Mux1/1 -> Reshape1/1
  Reshape1/1 -> [Dhat]
  [Dhat34] -> Gain1/1
  [basisSet] -> getDhat/1(psiz)  "basisSet"
  [es34] -> getDhat/2(es)
  getDhat/1(Dhat) -> [Dhat34]  "Dhat"
  Gain/1 -> Mux1/1
  Gain1/1 -> Mux1/2
  Constant/1 -> [Dhat12]
  Chebyshev Basis Functions/1(Tn) -> [Tnz]  "Tn"
  [x] -> Chebyshev Basis Functions/1(x)
  [tau] -> Chebyshev Basis Functions/2(tau)
  [Tnz] -> [basisSet]

== system simThreeLinkFTC/Controller/Disturbance Estimator/getx ==
  q : Inport
  qdot : Inport  Port=2
  H : Inport  Port=3
  Discrete Derivative : simulink/Discrete/Discrete Derivative  gainval=1.0  ICPrevScaledInput=0.0  InputProcessing=Inherited  OutMin=[]  OutMax=[]  OutDataType=fixdt(1, 16)  OutScaling=2^-10  RndMeth=Round  DoSatur=off
  Mux : Mux  Inputs=2
  Product6 : Product  Multiplication=Matrix(*)  RndMeth=Zero
  Reshape : Reshape  OutputDimensionality=Column vector (2-D)
  x : Outport
  xdot : Outport  Port=2
  wires:
  Discrete Derivative/1 -> xdot/1  "xdot"
  q/1 -> [q]
  qdot/1 -> [qdot]
  H/1 -> [H]
  [H] -> Product6/1
  [qdot] -> Product6/2
  Mux/1 -> Reshape/1
  Reshape/1 -> x/1, Discrete Derivative/1
  [q] -> Mux/1
  Product6/1 -> Mux/2

== system simThreeLinkFTC/Controller/Disturbance Estimator/getxhat ==
  Hinv : Inport
  tau : Inport  Port=2
  Cp : Inport  Port=3
  G : Inport  Port=4
  es : Inport  Port=5
  Dhat : Inport  Port=6
  Constant1 : Constant  Value=[eye(3,3)]  VectorParams1D=off
  Constant2 : Constant  Value=[zeros(3,3)]  VectorParams1D=off
  Constant3 : Constant  Value=[zeros(3,3)]
  Constant4 : Constant  Value=[zeros(3,1)]  VectorParams1D=off
  Constant5 : Constant  Value=As
  Discrete-Time Integrator : DiscreteIntegrator  IntegratorMethod=Integration: Backward Euler  InitialCondition=xhat0  InitialConditionSetting=State (most efficient)  SampleTime=-1  UpperSaturationLimit=Intmax  LowerSaturationLimit=Intmin
  Gain : Gain  Gain=-1
  Gain1 : Gain  Gain=-1
  Matrix Concatenate : Concatenate  Mode=Multidimensional array  ConcatenateDimension=2
  Matrix Concatenate1 : Concatenate  Mode=Multidimensional array
  Matrix Concatenate2 : Concatenate  Mode=Multidimensional array
  Matrix Concatenate3 : Concatenate  Mode=Multidimensional array  ConcatenateDimension=2
  Memory1 : Memory  X0=xhat0  InheritSampleTime=on  LinearizeMemory=on  LinearizeAsDelay=on
  Product1 : Product  Multiplication=Matrix(*)  RndMeth=Zero
  Product2 : Product  Multiplication=Matrix(*)  RndMeth=Zero
  Product6 : Product  Multiplication=Matrix(*)  RndMeth=Zero
  sum1 : Sum  Inputs=++++
  sum2 : Sum
  xhat : Outport
  xhatdot : Outport  Port=2
  wires:
  [Dhat] -> sum1/3  "Dhat"
  [B] -> sum1/2  "f"
  [Ax] -> sum1/1  "Ax"
  [Aes] -> sum1/4  "Aes"
  sum1/1 -> [xhatdot], Discrete-Time Integrator/1  "xhatdot"
  Discrete-Time Integrator/1 -> [xhat]  "xhat"
  Memory1/1 -> Product2/2
  Product2/1 -> [Ax]
  [xhat] -> Memory1/1
  Matrix Concatenate/1 -> Matrix Concatenate2/1
  Constant2/1 -> Matrix Concatenate/1
  Hinv/1 -> [Hinv]
  Matrix Concatenate2/1 -> Product2/1
  tau/1 -> [tau]
  Cp/1 -> [Cp]
  [G] -> Gain1/1
  [tau] -> sum2/2
  Constant4/1 -> Matrix Concatenate1/1
  sum2/1 -> Matrix Concatenate1/2
  Matrix Concatenate1/1 -> [B]
  Product6/1 -> [Aes]
  Constant5/1 -> Product6/1
  [es] -> Product6/2
  es/1 -> [es]
  Dhat/1 -> [Dhat]
  G/1 -> [G]
  Constant1/1 -> Matrix Concatenate/2
  Constant3/1 -> Matrix Concatenate3/1
  Matrix Concatenate3/1 -> Matrix Concatenate2/2
  [Hinv] -> Product1/1
  [Cp] -> Product1/2
  Product1/1 -> Gain/1
  Gain/1 -> Matrix Concatenate3/2
  Gain1/1 -> sum2/1
  [xhat] -> xhat/1
  [xhatdot] -> xhatdot/1

== system simThreeLinkFTC/Controller/FTC Controller/1st Link Compensator ==
  qc : Inport
  q : Inport  Port=2
  qdot : Inport  Port=3
  H : Inport  Port=4
  C : Inport  Port=5
  G : Inport  Port=6
  Enable : EnablePort
  " ADI Controller" : Subsystem  TreatAsAtomicUnit=on
  31-32 : Selector  NumberOfDimensions=2  InputPortWidth=3  IndexOptions=Index vector (dialog),Index vector (dialog)  Indices=3,[1 2]  OutputSizes=1,1
  33 : Selector  NumberOfDimensions=2  InputPortWidth=3  IndexOptions=Index vector (dialog),Index vector (dialog)  Indices=3,3  OutputSizes=1,1
  Add1 : Sum
  Constant : Constant  Value=0
  Gain3 : Gain  Gain=0
  Ground{,1..5} (6 alike) : Ground
  Memory : Memory  InheritSampleTime=on  LinearizeMemory=on  LinearizeAsDelay=on
  Mux : Mux  Inputs=2
  Partial FBL q2 Controller : Subsystem
  Product1 : Product  Multiplication=Matrix(*)  RndMeth=Zero
  Product5 : Product  Inputs=/  Multiplication=Matrix(*)  RndMeth=Zero
  Product6 : Product  Multiplication=Matrix(*)  RndMeth=Zero
  Reshape2 : Reshape  OutputDimensionality=Column vector (2-D)
  Select 12 : Selector  NumberOfDimensions=2  InputPortWidth=3  IndexOptions=Index vector (dialog),Index vector (dialog)  Indices=[2 3],1  OutputSizes=1,1
  Terminator : Terminator
  Terminator1 : Terminator
  tau : Outport
  wires:
  Select 12/1 -> [qc]
  [compensation] -> Terminator1/1
  [Hp] -> 33/1, 31-32/1
  31-32/1 -> [H12]
  33/1 -> [H11]
  Mux/1 -> Reshape2/1
  [tau] -> Mux/2
  Constant/1 -> Mux/1
  Reshape2/1 -> tau/1  "tau"
  G/1 -> [Gp]
  C/1 -> [Cp]
  H/1 -> [Hp]
  Partial FBL q2 Controller/1(tau) -> [tau]  "tau_q2"
  Ground5/1 -> " ADI Controller"/4(Comp)
  Memory/1 -> [compensation]
  Gain3/1 -> Memory/1
  [v] -> Product1/2
  Product6/1 -> Product1/1
  Product1/1 -> Gain3/1
  [H12] -> Product6/2
  Product5/1 -> Product6/1
  [H11] -> Product5/1
  Ground1/1 -> Partial FBL q2 Controller/2(qcdot)
  Partial FBL q2 Controller/2(v) -> [v]
  [Gp] -> Partial FBL q2 Controller/7(G)
  [Cp] -> Partial FBL q2 Controller/6(C)
  [Hp] -> Partial FBL q2 Controller/5(H)
  [qdot] -> Partial FBL q2 Controller/4(qdot)
  [q] -> Partial FBL q2 Controller/3(q)
  Add1/1 -> Partial FBL q2 Controller/1(qc)
  [qc] -> Add1/1
  Ground/1 -> Add1/2
  " ADI Controller"/1(r) -> Terminator/1  "r"
  Ground4/1 -> " ADI Controller"/3(qdot)
  Ground3/1 -> " ADI Controller"/2(q)
  Ground2/1 -> " ADI Controller"/1(qc)
  qc/1 -> Select 12/1  "ftc_qc"
  qdot/1 -> [qdot]
  q/1 -> [q]

== system simThreeLinkFTC/Controller/FTC Controller/3rd Link Compensator ==
  qc : Inport
  q : Inport  Port=2
  qdot : Inport  Port=3
  H : Inport  Port=4
  C : Inport  Port=5
  G : Inport  Port=6
  Enable : EnablePort
  " ADI Controller" : Subsystem  TreatAsAtomicUnit=on
  31-32 : Selector  NumberOfDimensions=2  InputPortWidth=3  IndexOptions=Index vector (dialog),Index vector (dialog)  Indices=3,[1 2]  OutputSizes=1,1
  33 : Selector  NumberOfDimensions=2  InputPortWidth=3  IndexOptions=Index vector (dialog),Index vector (dialog)  Indices=3,3  OutputSizes=1,1
  Add1 : Sum
  Constant : Constant  Value=0
  Gain1 : Gain  Gain="[0  ; 1]"
  Gain2 : Gain  Gain="[0  ; 1]"
  Gain3 : Gain  Gain=[0 -1]'
  Memory : Memory  InheritSampleTime=on  LinearizeMemory=on  LinearizeAsDelay=on
  Mux : Mux  Inputs=2
  Partial FBL q2 Controller : Subsystem
  Product1 : Product  Multiplication=Matrix(*)  RndMeth=Zero
  Product5 : Product  Inputs=/  Multiplication=Matrix(*)  RndMeth=Zero
  Product6 : Product  Multiplication=Matrix(*)  RndMeth=Zero
  Reshape2 : Reshape  OutputDimensionality=Column vector (2-D)
  Select 1-1 : Selector  InputPortWidth=2
  Select 1-2 : Selector  NumberOfDimensions=2  InputPortWidth=3  IndexOptions=Index vector (dialog),Index vector (dialog)  Indices=[1 2],1  OutputSizes=1,1
  Select 1-3 : Selector  InputPortWidth=2  Indices=2
  tau : Outport
  wires:
  q/1 -> [q]
  qdot/1 -> [qdot]
  [q] -> " ADI Controller"/2(q)
  [qdot] -> " ADI Controller"/3(qdot)
  " ADI Controller"/1(r) -> [r]  "r"
  [qc] -> Select 1-2/1
  Add1/1 -> Partial FBL q2 Controller/1(qc)
  [q] -> Partial FBL q2 Controller/3(q)
  [qdot] -> Partial FBL q2 Controller/4(qdot)
  [Hp] -> Partial FBL q2 Controller/5(H)
  [Cp] -> Partial FBL q2 Controller/6(C)
  [Gp] -> Partial FBL q2 Controller/7(G)
  Partial FBL q2 Controller/2(v) -> [v]
  [H11] -> Product5/1
  Product5/1 -> Product6/1
  [H12] -> Product6/2
  Product1/1 -> Gain3/1
  Product6/1 -> Product1/1
  [v] -> Product1/2
  Gain3/1 -> Memory/1
  Memory/1 -> [compensation]
  Partial FBL q2 Controller/1(tau) -> [tau]  "tau_q2"
  H/1 -> [Hp]
  C/1 -> [Cp]
  G/1 -> [Gp]
  Reshape2/1 -> tau/1  "tau"
  Mux/1 -> Reshape2/1
  33/1 -> [H11]
  31-32/1 -> [H12]
  [Hp] -> 31-32/1, 33/1
  Constant/1 -> Mux/2
  [tau] -> Mux/1
  Select 1-2/1 -> Add1/1
  qc/1 -> [qc]  "ftc_qc"
  [qc] -> " ADI Controller"/1(qc)
  [compensation] -> " ADI Controller"/4(Comp)
  [r] -> Select 1-1/1
  [r] -> Select 1-3/1
  Gain2/1 -> Add1/2
  Select 1-1/1 -> Gain2/1
  Select 1-3/1 -> Gain1/1
  Gain1/1 -> Partial FBL q2 Controller/2(qcdot)

== system simThreeLinkFTC/Controller/Fault Detection/Triggered step ==
  Trigger : TriggerPort  PortDimensions=1
  Constant : Constant
  Out1 : Outport  InitialOutput=0
  wires:
  Constant/1 -> Out1/1

== system simThreeLinkFTC/Controller/Get System Parameters/get Plant Parameters ==
  H : Inport
  C : Inport  Port=2
  G : Inport  Port=3
  qdot : Inport  Port=4
  Cprime : Inport  Port=5
  {1,5,7,11} (4 alike) : Selector  NumberOfDimensions=2  InputPortWidth=3  IndexOptions=Index vector (dialog),Index vector (dialog)  Indices=1,1  OutputSizes=1,1
  12 : Selector  NumberOfDimensions=2  InputPortWidth=3  IndexOptions=Index vector (dialog),Index vector (dialog)  Indices=1,2  OutputSizes=1,1
  2 : Selector  NumberOfDimensions=2  InputPortWidth=3  IndexOptions=Index vector (dialog),Index vector (dialog)  Indices=1,2  OutputSizes=1,1
  {3,6,8,21} (4 alike) : Selector  NumberOfDimensions=2  InputPortWidth=3  IndexOptions=Index vector (dialog),Index vector (dialog)  Indices=2,1  OutputSizes=1,1
  22 : Selector  NumberOfDimensions=2  InputPortWidth=3  IndexOptions=Index vector (dialog),Index vector (dialog)  Indices=2,2  OutputSizes=1,1
  4 : Selector  NumberOfDimensions=2  InputPortWidth=3  IndexOptions=Index vector (dialog),Index vector (dialog)  Indices=2,2  OutputSizes=1,1
  Bus Creator : BusCreator  Inputs=16
  Product5 : Product  Multiplication=Matrix(*)  RndMeth=Zero
  Sum of Elements1 : Sum
  busData : Outport
  wires:
  [H] -> 11/1, 12/1, 21/1, 22/1
  [C] -> 1/1, 2/1, 4/1, 3/1
  [G] -> 6/1, 5/1
  [C] -> Product5/1
  [qdot] -> Product5/2
  Product5/1 -> Sum of Elements1/1
  [G] -> Sum of Elements1/2
  Sum of Elements1/1 -> 7/1, 8/1
  Bus Creator/1 -> busData/1
  H/1 -> [H]  "H"
  C/1 -> [C]  "C"
  G/1 -> [G]  "G"
  qdot/1 -> [qdot]
  [G] -> Bus Creator/4
  [Cprime] -> Bus Creator/3
  [C] -> Bus Creator/2
  [H] -> Bus Creator/1
  22/1 -> Bus Creator/8  "H22"
  21/1 -> Bus Creator/7  "H21"
  1/1 -> Bus Creator/9  "C11"
  12/1 -> Bus Creator/6  "H12"
  2/1 -> Bus Creator/10  "C12"
  11/1 -> Bus Creator/5  "H11"
  3/1 -> Bus Creator/11  "C21"
  4/1 -> Bus Creator/12  "C22"
  5/1 -> Bus Creator/13  "G_1"
  6/1 -> Bus Creator/14  "G_2"
  7/1 -> Bus Creator/15  "phi1"
  8/1 -> Bus Creator/16  "phi2"
  Cprime/1 -> [Cprime]  "Cprime"

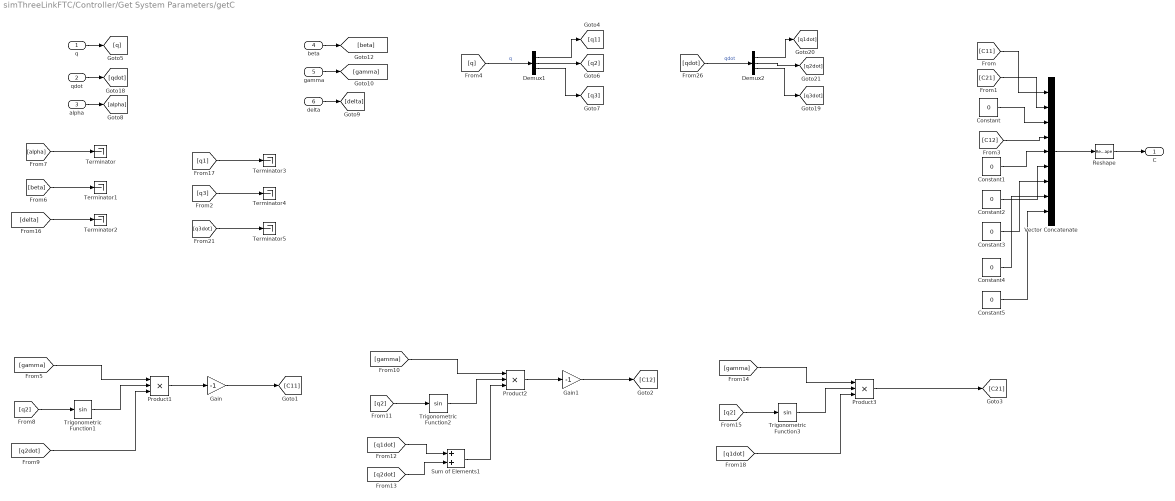
== system simThreeLinkFTC/Controller/Get System Parameters/getC ==
  q : Inport
  qdot : Inport  Port=2
  alpha : Inport  Port=3
  beta : Inport  Port=4
  gamma : Inport  Port=5
  delta : Inport  Port=6
  Constant{,1..5} (6 alike) : Constant  Value=0  VectorParams1D=off
  Demux1 : Demux  Outputs=3
  Demux2 : Demux  Outputs=3
  Gain : Gain  Gain=-1
  Gain1 : Gain  Gain=-1
  Product1 : Product  Inputs=3
  Product2 : Product  Inputs=3
  Product3 : Product  Inputs=3
  Reshape : Reshape  OutputDimensionality=Customize  OutputDimensions=[3,3]
  Sum of Elements1 : Sum
  Terminator{,1..5} (6 alike) : Terminator
  Trigonometric Function1 : Trigonometry
  Trigonometric Function2 : Trigonometry
  Trigonometric Function3 : Trigonometry
  Vector Concatenate : Concatenate  NumInputs=9
  C : Outport
  wires:
  [C11] -> Vector Concatenate/1
  [C21] -> Vector Concatenate/2
  Constant/1 -> Vector Concatenate/3
  Constant1/1 -> Vector Concatenate/5
  [C12] -> Vector Concatenate/4
  Vector Concatenate/1 -> Reshape/1
  beta/1 -> [beta]
  gamma/1 -> [gamma]
  delta/1 -> [delta]
  alpha/1 -> [alpha]
  Demux1/2 -> [q2]
  Demux1/3 -> [q3]
  Demux1/1 -> [q1]
  [q] -> Demux1/1  "q"
  q/1 -> [q]
  Reshape/1 -> C/1
  qdot/1 -> [qdot]
  [qdot] -> Demux2/1  "qdot"
  Demux2/1 -> [q1dot]
  Demux2/3 -> [q3dot]
  Demux2/2 -> [q2dot]
  Constant2/1 -> Vector Concatenate/6
  Constant3/1 -> Vector Concatenate/7
  Constant4/1 -> Vector Concatenate/8
  Constant5/1 -> Vector Concatenate/9
  [q3dot] -> Terminator5/1
  [q3] -> Terminator4/1
  [q1] -> Terminator3/1
  [alpha] -> Terminator/1
  [beta] -> Terminator1/1
  [delta] -> Terminator2/1
  [q2] -> Trigonometric Function1/1
  [gamma] -> Product1/1
  Trigonometric Function1/1 -> Product1/2
  [q2dot] -> Product1/3
  Product1/1 -> Gain/1
  Gain/1 -> [C11]
  [q2] -> Trigonometric Function2/1
  [gamma] -> Product2/1
  Trigonometric Function2/1 -> Product2/2
  Product2/1 -> Gain1/1
  Gain1/1 -> [C12]
  [q1dot] -> Sum of Elements1/1
  [q2dot] -> Sum of Elements1/2
  Sum of Elements1/1 -> Product2/3
  [q2] -> Trigonometric Function3/1
  [gamma] -> Product3/1
  Trigonometric Function3/1 -> Product3/2
  [q1dot] -> Product3/3
  Product3/1 -> [C21]

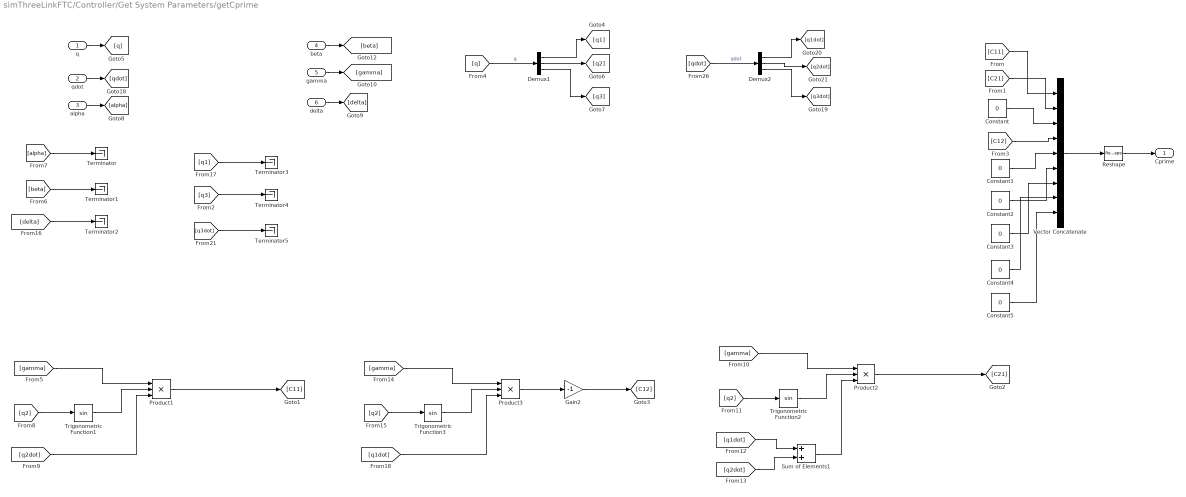
== system simThreeLinkFTC/Controller/Get System Parameters/getCprime ==
  q : Inport
  qdot : Inport  Port=2
  alpha : Inport  Port=3
  beta : Inport  Port=4
  gamma : Inport  Port=5
  delta : Inport  Port=6
  Constant{,1..5} (6 alike) : Constant  Value=0  VectorParams1D=off
  Demux1 : Demux  Outputs=3
  Demux2 : Demux  Outputs=3
  Gain2 : Gain  Gain=-1
  Product1 : Product  Inputs=3
  Product2 : Product  Inputs=3
  Product3 : Product  Inputs=3
  Reshape : Reshape  OutputDimensionality=Customize  OutputDimensions=[3,3]
  Sum of Elements1 : Sum
  Terminator{,1..5} (6 alike) : Terminator
  Trigonometric Function1 : Trigonometry
  Trigonometric Function2 : Trigonometry
  Trigonometric Function3 : Trigonometry
  Vector Concatenate : Concatenate  NumInputs=9
  Cprime : Outport
  wires:
  Product3/1 -> Gain2/1
  [q1dot] -> Product3/3
  Trigonometric Function3/1 -> Product3/2
  [gamma] -> Product3/1
  [q2] -> Trigonometric Function3/1
  Sum of Elements1/1 -> Product2/3
  [q2dot] -> Sum of Elements1/2
  [q1dot] -> Sum of Elements1/1
  Product2/1 -> [C21]
  Trigonometric Function2/1 -> Product2/2
  [gamma] -> Product2/1
  [q2] -> Trigonometric Function2/1
  Product1/1 -> [C11]
  [q2dot] -> Product1/3
  Trigonometric Function1/1 -> Product1/2
  [gamma] -> Product1/1
  [q2] -> Trigonometric Function1/1
  [delta] -> Terminator2/1
  [beta] -> Terminator1/1
  [alpha] -> Terminator/1
  [q1] -> Terminator3/1
  [q3] -> Terminator4/1
  [q3dot] -> Terminator5/1
  Constant5/1 -> Vector Concatenate/9
  Constant4/1 -> Vector Concatenate/8
  Constant3/1 -> Vector Concatenate/7
  Constant2/1 -> Vector Concatenate/6
  Demux2/2 -> [q2dot]
  Demux2/3 -> [q3dot]
  Demux2/1 -> [q1dot]
  [qdot] -> Demux2/1  "qdot"
  qdot/1 -> [qdot]
  Reshape/1 -> Cprime/1
  q/1 -> [q]
  [q] -> Demux1/1  "q"
  Demux1/1 -> [q1]
  Demux1/3 -> [q3]
  Demux1/2 -> [q2]
  alpha/1 -> [alpha]
  delta/1 -> [delta]
  gamma/1 -> [gamma]
  beta/1 -> [beta]
  Vector Concatenate/1 -> Reshape/1
  [C12] -> Vector Concatenate/4
  Constant1/1 -> Vector Concatenate/5
  Constant/1 -> Vector Concatenate/3
  [C21] -> Vector Concatenate/2
  [C11] -> Vector Concatenate/1
  Gain2/1 -> [C12]

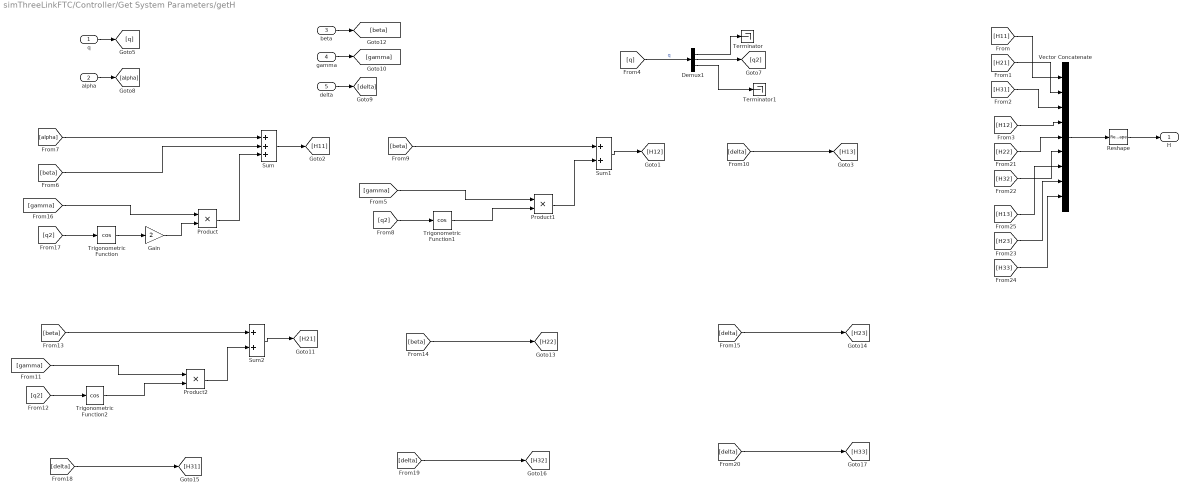
== system simThreeLinkFTC/Controller/Get System Parameters/getH ==
  q : Inport
  alpha : Inport  Port=2
  beta : Inport  Port=3
  gamma : Inport  Port=4
  delta : Inport  Port=5
  Demux1 : Demux  Outputs=3
  Gain : Gain  Gain=2
  Product : Product
  Product1 : Product
  Product2 : Product
  Reshape : Reshape  OutputDimensionality=Customize  OutputDimensions=[3,3]
  Sum : Sum  Inputs=+++
  Sum1 : Sum
  Sum2 : Sum
  Terminator : Terminator
  Terminator1 : Terminator
  Trigonometric Function : Trigonometry  Operator=cos
  Trigonometric Function1 : Trigonometry  Operator=cos
  Trigonometric Function2 : Trigonometry  Operator=cos
  Vector Concatenate : Concatenate  NumInputs=9
  H : Outport
  wires:
  Reshape/1 -> H/1
  Sum/1 -> [H11]
  q/1 -> [q]
  [q] -> Demux1/1  "q"
  Demux1/1 -> Terminator/1
  Demux1/2 -> [q2]
  alpha/1 -> [alpha]
  delta/1 -> [delta]
  gamma/1 -> [gamma]
  beta/1 -> [beta]
  [q2] -> Trigonometric Function/1
  Trigonometric Function/1 -> Gain/1
  [gamma] -> Product/1
  Gain/1 -> Product/2
  [alpha] -> Sum/1
  [beta] -> Sum/2
  Product/1 -> Sum/3
  Sum1/1 -> [H12]
  [q2] -> Trigonometric Function1/1
  [gamma] -> Product1/1
  Trigonometric Function1/1 -> Product1/2
  [beta] -> Sum1/1
  Product1/1 -> Sum1/2
  [delta] -> [H13]
  Sum2/1 -> [H21]
  [q2] -> Trigonometric Function2/1
  [gamma] -> Product2/1
  Trigonometric Function2/1 -> Product2/2
  [beta] -> Sum2/1
  Product2/1 -> Sum2/2
  [beta] -> [H22]
  [delta] -> [H23]
  [delta] -> [H31]
  [delta] -> [H32]
  [delta] -> [H33]
  Vector Concatenate/1 -> Reshape/1
  [H12] -> Vector Concatenate/4
  [H22] -> Vector Concatenate/5
  [H31] -> Vector Concatenate/3
  [H32] -> Vector Concatenate/6
  [H21] -> Vector Concatenate/2
  [H11] -> Vector Concatenate/1
  [H13] -> Vector Concatenate/7
  [H23] -> Vector Concatenate/8
  [H33] -> Vector Concatenate/9
  Demux1/3 -> Terminator1/1

== system simThreeLinkFTC/Controller/Nominal Controller/FBL Controller ==
  r : Inport
  q : Inport  Port=2
  qdot : Inport  Port=3
  H : Inport  Port=4
  Phi : Inport  Port=5
  Add : Sum  Inputs=-+
  Add1 : Sum  Inputs=-+
  Add2 : Sum
  Add3 : Sum
  Add4 : Sum
  Constant2 : Constant  Value=[0 0 0]'
  Discrete Derivative : simulink/Discrete/Discrete Derivative  gainval=1.0  ICPrevScaledInput=0.0  InputProcessing=Inherited  OutMin=[]  OutMax=[]  OutDataType=fixdt(1, 16)  OutScaling=2^-10  DoSatur=off
  Gain : Gain  Gain=-Kv
  Gain1 : Gain  Gain=-Kp
  Product2 : Product  Multiplication=Matrix(*)  RndMeth=Zero
  Saturation : Saturate  UpperLimit=10  LowerLimit=-10
  tau : Outport
  wires:
  [v] -> Product2/2
  Product2/1 -> Add4/1
  [Phi] -> Add4/2
  [H] -> Product2/1
  [r] -> Add/1
  Add/1 -> [e]  "e"
  Discrete Derivative/1 -> Saturation/1
  [qdot] -> Add1/2
  Add1/1 -> [edot]  "edot"
  [edot] -> Gain/1
  Constant2/1 -> Add2/1
  Gain/1 -> Add2/2
  [e] -> Gain1/1
  Add2/1 -> Add3/1
  Gain1/1 -> Add3/2
  Add3/1 -> [v]  "v"
  [q] -> Add/2
  [r] -> Discrete Derivative/1
  Saturation/1 -> Add1/1
  r/1 -> [r]  "r"
  Phi/1 -> [Phi]
  H/1 -> [H]
  Add4/1 -> tau/1  "tau"
  q/1 -> [q]
  qdot/1 -> [qdot]

== system simThreeLinkFTC/System/System Parameters/get Plant Parameters ==
  H : Inport
  C : Inport  Port=2
  G : Inport  Port=3
  qdot : Inport  Port=4
  alpha : Inport  Port=5
  beta : Inport  Port=6
  gamma : Inport  Port=7
  delta : Inport  Port=8
  7 : Selector  NumberOfDimensions=2  InputPortWidth=3  IndexOptions=Index vector (dialog),Index vector (dialog)  Indices=1,1  OutputSizes=1,1
  8 : Selector  NumberOfDimensions=2  InputPortWidth=3  IndexOptions=Index vector (dialog),Index vector (dialog)  Indices=2,1  OutputSizes=1,1
  9 : Selector  NumberOfDimensions=2  InputPortWidth=3  IndexOptions=Index vector (dialog),Index vector (dialog)  Indices=3,1  OutputSizes=1,1
  Bus Creator : BusCreator  Inputs=10
  Product5 : Product  Multiplication=Matrix(*)  RndMeth=Zero
  Sum of Elements1 : Sum
  busData : Outport
  wires:
  [C] -> Product5/1
  [qdot] -> Product5/2
  Product5/1 -> Sum of Elements1/1
  [G] -> Sum of Elements1/2
  Sum of Elements1/1 -> 7/1, 9/1, 8/1
  Bus Creator/1 -> busData/1
  H/1 -> [H]  "H"
  C/1 -> [C]  "C"
  G/1 -> [G]  "G"
  qdot/1 -> [qdot]
  [G] -> Bus Creator/3
  [C] -> Bus Creator/2
  [H] -> Bus Creator/1
  beta/1 -> [beta]
  gamma/1 -> [gamma]
  delta/1 -> [delta]
  alpha/1 -> [alpha]
  7/1 -> Bus Creator/4  "phi1"
  8/1 -> Bus Creator/5  "phi2"
  9/1 -> Bus Creator/6  "phi3"
  [alpha] -> Bus Creator/7  "alpha"
  [beta] -> Bus Creator/8  "beta"
  [gamma] -> Bus Creator/9  "gamma"
  [delta] -> Bus Creator/10  "delta"

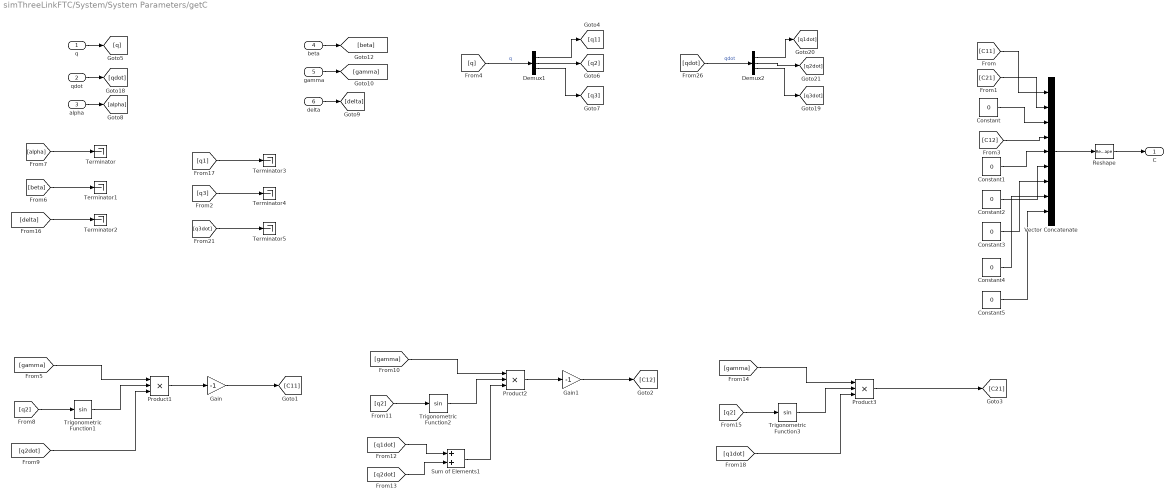
== system simThreeLinkFTC/System/System Parameters/getC ==
  q : Inport
  qdot : Inport  Port=2
  alpha : Inport  Port=3
  beta : Inport  Port=4
  gamma : Inport  Port=5
  delta : Inport  Port=6
  Constant{,1..5} (6 alike) : Constant  Value=0  VectorParams1D=off
  Demux1 : Demux  Outputs=3
  Demux2 : Demux  Outputs=3
  Gain : Gain  Gain=-1
  Gain1 : Gain  Gain=-1
  Product1 : Product  Inputs=3
  Product2 : Product  Inputs=3
  Product3 : Product  Inputs=3
  Reshape : Reshape  OutputDimensionality=Customize  OutputDimensions=[3,3]
  Sum of Elements1 : Sum
  Terminator{,1..5} (6 alike) : Terminator
  Trigonometric Function1 : Trigonometry
  Trigonometric Function2 : Trigonometry
  Trigonometric Function3 : Trigonometry
  Vector Concatenate : Concatenate  NumInputs=9
  C : Outport
  wires:
  [C11] -> Vector Concatenate/1
  [C21] -> Vector Concatenate/2
  Constant/1 -> Vector Concatenate/3
  Constant1/1 -> Vector Concatenate/5
  [C12] -> Vector Concatenate/4
  Vector Concatenate/1 -> Reshape/1
  beta/1 -> [beta]
  gamma/1 -> [gamma]
  delta/1 -> [delta]
  alpha/1 -> [alpha]
  Demux1/2 -> [q2]
  Demux1/3 -> [q3]
  Demux1/1 -> [q1]
  [q] -> Demux1/1  "q"
  q/1 -> [q]
  Reshape/1 -> C/1
  qdot/1 -> [qdot]
  [qdot] -> Demux2/1  "qdot"
  Demux2/1 -> [q1dot]
  Demux2/3 -> [q3dot]
  Demux2/2 -> [q2dot]
  Constant2/1 -> Vector Concatenate/6
  Constant3/1 -> Vector Concatenate/7
  Constant4/1 -> Vector Concatenate/8
  Constant5/1 -> Vector Concatenate/9
  [q3dot] -> Terminator5/1
  [q3] -> Terminator4/1
  [q1] -> Terminator3/1
  [alpha] -> Terminator/1
  [beta] -> Terminator1/1
  [delta] -> Terminator2/1
  [q2] -> Trigonometric Function1/1
  [gamma] -> Product1/1
  Trigonometric Function1/1 -> Product1/2
  [q2dot] -> Product1/3
  Product1/1 -> Gain/1
  Gain/1 -> [C11]
  [q2] -> Trigonometric Function2/1
  [gamma] -> Product2/1
  Trigonometric Function2/1 -> Product2/2
  Product2/1 -> Gain1/1
  Gain1/1 -> [C12]
  [q1dot] -> Sum of Elements1/1
  [q2dot] -> Sum of Elements1/2
  Sum of Elements1/1 -> Product2/3
  [q2] -> Trigonometric Function3/1
  [gamma] -> Product3/1
  Trigonometric Function3/1 -> Product3/2
  [q1dot] -> Product3/3
  Product3/1 -> [C21]
